simulink model "Checkpoint1"  (R2024a)
settings: Solver=VariableStepAuto  StartTime=0.0  StopTime=10.0  MaxStep=1e-3  RelTol=1e-3
libraries: simulink x1

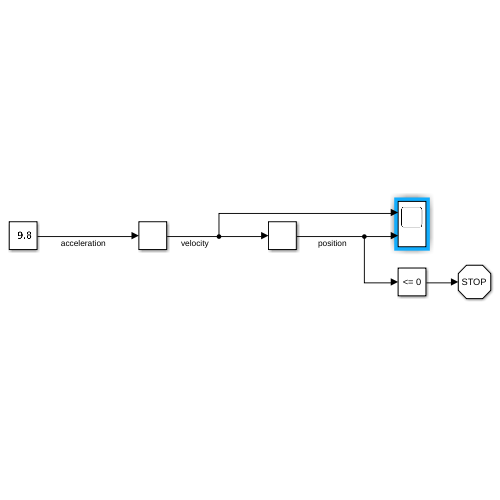
[thumbnail: Simulink's stored preview of the top-level diagram]
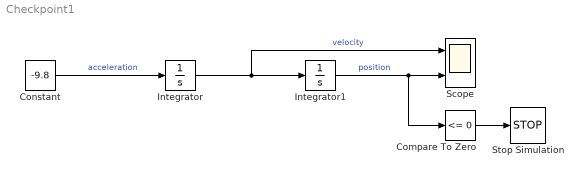
== system Checkpoint1 ==
  Compare To Zero : simulink/Logic and Bit Operations/Compare To Zero  relop=<=  OutDataTypeStr=boolean
  Constant : Constant  Value=-9.8
  Integrator : Integrator  InitialCondition=0.5
  Integrator1 : Integrator  InitialCondition=1
  Scope : Scope  NumInputPorts=2
  Stop Simulation : Stop
  wires:
  Constant/1 -> Integrator/1  "acceleration"
  Integrator/1 -> Scope/1, Integrator1/1  "velocity"
  Integrator1/1 -> Compare To Zero/1, Scope/2  "position"
  Compare To Zero/1 -> Stop Simulation/1
